simulink model "Ts2"  (R2024b)
settings: Solver=VariableStepAuto  StartTime=0.0  StopTime=20  RelTol=1e-3
values from neighbouring files (symbols this model uses):
  A = [ -1.2 -1.40 ; -0.05 -1]    [tema1.m]
  B = [ 1.2 -8.005 ; 1 -1.7]    [tema1.m]
  C = [-Ti 0 ; 0 -1.3]    [tema1.m]
  D = [0 0 ; 0 0]    [tema1.m]
settings Model: Creator=albertrosca  LastModifiedBy=albertrosca

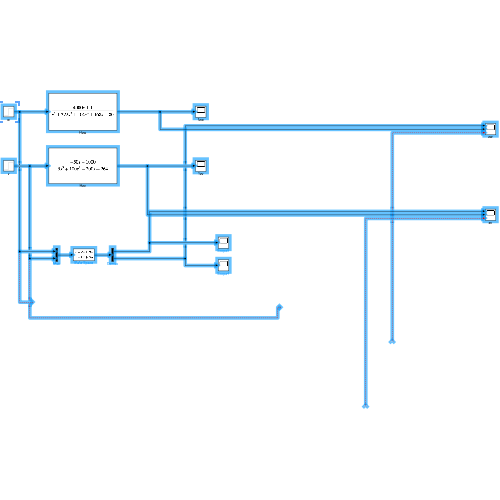
[thumbnail: Simulink's stored preview of the top-level diagram]
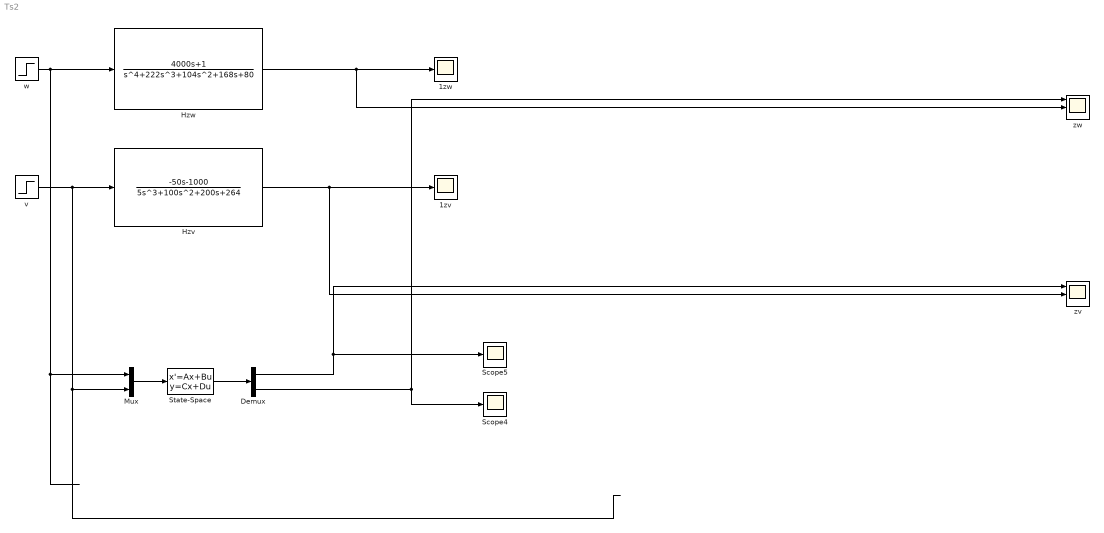
== system Ts2 ==
  1zv : Scope
  1zw : Scope
  Demux : Demux  Outputs=2
  Hzv : TransferFcn  Numerator=[-50 -1000]  Denominator=[5 100 200 264]
  Hzw : TransferFcn  Numerator=[4000 1]  Denominator=[1 222 104 168 80]
  Mux : Mux  Inputs=2
  Scope4 : Scope
  Scope5 : Scope
  State-Space : StateSpace  A=A  B=B  C=C  D=D  InitialCondition=0
  v : Step  Time=5  After=10  SampleTime=0
  w : Step  Time=3  After=6  SampleTime=0
  zv : Scope  NumInputPorts=3
  zw : Scope  NumInputPorts=3
  wires:
  ? -> zw/3
  ? -> zv/3
  Demux/2 -> zw/1, Scope4/1
  State-Space/1 -> Demux/1
  Demux/1 -> zv/1, Scope5/1
  Mux/1 -> State-Space/1
  Hzw/1 -> zw/2, 1zw/1
  v/1 -> Mux/2, Hzv/1
  w/1 -> Mux/1, Hzw/1
  Hzv/1 -> zv/2, 1zv/1
